simulink model "model_z_funkcja"  (R2019b)
settings: Solver=FixedStepAuto  StartTime=0.0  StopTime=0.01  RelTol=1e-3
libraries: hdlsllib x1
settings Model: Creator=bwieczorek  LastModifiedBy=bwieczorek
settings OptimizationCC: BlockReduction=off  ConditionallyExecuteInputs=off
settings DebuggingCC: SignalRangeChecking=warning

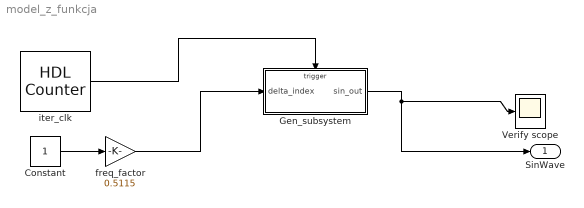
== system model_z_funkcja ==
  Constant : Constant
  Gen_subsystem : Subsystem  TreatAsAtomicUnit=on
  Verify scope : Scope
  freq_factor : Gain  Gain=0.5115  OutDataTypeStr=Inherit: Same as input
  iter_clk : hdlsllib/Sources/HDL Counter  CountType=Count limited  CountInit=0  CountStep=1  CountMax=1  CountFromType=Initial value  CountFrom=0  CountResetPort=off  CountLoadPort=off  CountEnbPort=off  CountDirPort=off  CountDataType=Unsigned  CountWordLen=1  CountFracLen=0  CountSampTime=1e-6
      settings: SourceProductName=Simulink
  SinWave : Outport  VectorParamsAs1DForOutWhenUnconnected=off
  wires:
  Gen_subsystem/1(sin_out) -> SinWave/1, Verify scope/1
  iter_clk/1 -> Gen_subsystem/Trigger
  freq_factor/1 -> Gen_subsystem/1(delta_index)
  Constant/1 -> freq_factor/1

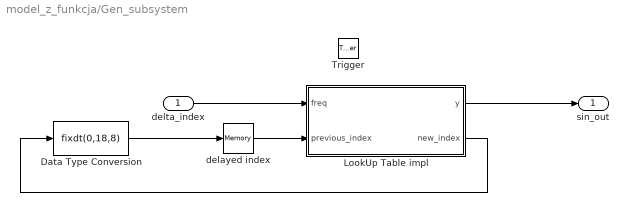
== system model_z_funkcja/Gen_subsystem ==
  delta_index : Inport
  Trigger : TriggerPort  VariantControl=Variant  InitialTriggerSignalState=zero
  Data Type Conversion : DataTypeConversion  OutDataTypeStr=fixdt(0,18,8)
  LookUp Table impl : MATLAB Function  TreatAsAtomicUnit=on
  delayed index : Memory  InheritSampleTime=on
  sin_out : Outport  InitialOutput=[0]
  wires:
  delayed index/1 -> LookUp Table impl/2(previous_index)
  delta_index/1 -> LookUp Table impl/1(freq)
  LookUp Table impl/1(y) -> sin_out/1
  LookUp Table impl/2(new_index) -> Data Type Conversion/1
  Data Type Conversion/1 -> delayed index/1

== matlab function model_z_funkcja/Gen_subsystem/LookUp Table impl ==
  data: freq input; y output; previous_index input fixdt(0,18,8); new_index output fixdt(0,19,8)
function [y, new_index]= fcn(freq, previous_index)
%#codegen
loader = coder.load('tableSin.mat');
table = loader.tableSin;
new_index = fi(previous_index + freq, 0, 19, 8);
if(new_index >= 256)  %check if index overflows the table
new_index = fi(new_index - fi(256,0,9,0),0,19,8);    
end
if(mod(new_index, fi(1,0,1,0)) == 0 )%check if index is int
y = fi(table((mod(new_index,fi(256,0,9,0)))+1),1,18,17); 
else
index_floor = floor(new_index);
if(index_floor == 255)  %check if ceil value overflows the table
index_ceil = fi(0,0,12,0); 
else
index_ceil = ceil(new_index);    
end
sin_floor = table(index_floor+1);
sin_ceil = table(index_ceil+1);
a = sin_ceil - sin_floor;
y = fi(a*mod(new_index,fi(1,0,1,0)) + sin_floor, 1, 18, 17); 
end
